simulink model "msdMultipleFreq"  (R2020b)
settings: Solver=VariableStepAuto  StartTime=0.0  StopTime=40  RelTol=1e-6
undefined symbols (not defined in the file): c, F, k, m, x_0, x_dot_0
settings Model: Creator=Rocksmithed  LastModifiedBy=Rocksmithed
settings DataIOCC: SaveFormat=Array
settings HardwareCC: TargetBitPerPointer=64  TargetBitPerSizeT=64  TargetBitPerPtrDiffT=64  TargetLongLongMode=on  TargetIntDivRoundTo=Zero  TargetEndianess=LittleEndian  TargetWordSize=64  TargetHWDeviceType=MATLAB Host  ProdEqTarget=off
settings RTWCC: Description=Rapid Simulation Target  SystemTargetFile=rsim.tlc  TemplateMakefile=rsim_default_tmf
settings RSimTargetCC: TargetLangStandard=C99 (ISO)

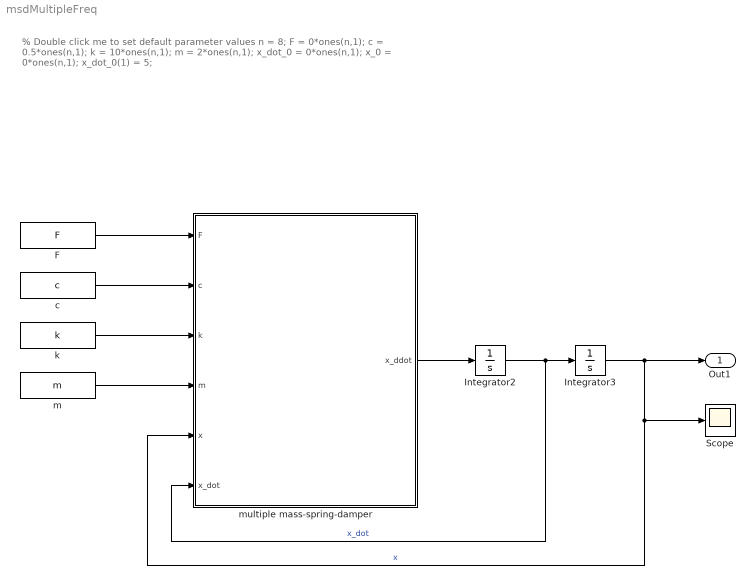
== system msdMultipleFreq ==
  note: % Double click me to set default parameter values
      | n = 8;
      | F = 0*ones(n,1);
      | c = 0.5*ones(n,1);
      | k = 10*ones(n,1);
      | m = 2*ones(n,1);
      | x_dot_0 = 0*ones(n,1);
      | x_0 = 0*ones(n,1);
      | x_dot_0(1) = 5;
  F : Constant  Value=F
  Integrator2 : Integrator  InitialCondition=x_dot_0
  Integrator3 : Integrator  InitialCondition=x_0
  Scope : Scope
  c : Constant  Value=c
  k : Constant  Value=k
  m : Constant  Value=m
  multiple mass-spring-damper : MATLAB Function  TreatAsAtomicUnit=on
  Out1 : Outport
  wires:
  Integrator2/1 -> multiple mass-spring-damper/6(x_dot), Integrator3/1  "x_dot"
  F/1 -> multiple mass-spring-damper/1(F)
  c/1 -> multiple mass-spring-damper/2(c)
  k/1 -> multiple mass-spring-damper/3(k)
  m/1 -> multiple mass-spring-damper/4(m)
  multiple mass-spring-damper/1(x_ddot) -> Integrator2/1
  Integrator3/1 -> multiple mass-spring-damper/5(x), Scope/1, Out1/1  "x"

== matlab function msdMultipleFreq/multiple mass-spring-damper ==
  data: F input; x_ddot output; c input; k input; m input; x input; x_dot input
function x_ddot = multipleMassSpringDamper(F, c, k, m, x, x_dot)
%#codegen

n = 8;

x_ddot = zeros(n,1);

x_ddot(1) = -(-F(1)+c(1).*x_dot(1)+k(1).*x(1)+c(2).*(x_dot(1)-x_dot(2))+k(2).*(x(1)-x(2)))./m(1);
if (n > 2)
    x_ddot(2:n-1) = F(2:n-1) + k(3:n).*( x(3:n) - x(2:n-1) ) + c(3:n).*( x_dot(3:n) - x_dot(2:n-1) )...
                             - k(2:n-1).*( x(2:n-1) - x(1:n-2) ) - c(2:n-1).*( x_dot(2:n-1) - x_dot(1:n-2) );
end
x_ddot(n) = (F(n)-c(n).*(x_dot(n)-x_dot(n-1))-k(n).*(x(n)-x(n-1)))./m(n) ;
